simulink model "visual_servoing"  (R2023a)
settings: Solver=ode2  StartTime=0.0  StopTime=inf  FixedStep=1/30  RelTol=1e-3  EnableMultiTasking=on
undefined symbols (not defined in the file): gcbh, height, HIL, JPEG, left, qc_get_step_size, top, video_display_show, width
libraries: quarc_library x21, simulink x4
settings Model: ExtModeTrigDuration=10000  Creator=msaravanan  LastModifiedBy=msaravanan
settings SolverCC: AlgebraicLoopSolver=TrustRegion  PositivePriorityOrder=on
settings DataIOCC: ReturnWorkspaceOutputs=off
settings DebuggingCC: UnconnectedInputMsg=warning  UnconnectedOutputMsg=warning  UnconnectedLineMsg=warning  ArithmeticOperatorsInVariantConditions=warning
settings ModelReferenceCC: EnableRefExpFcnMdlSchedulingChecks=on
settings SFSimCC: SimUseLocalCustomCode=off  CustomCodeUndefinedFunction=UseInterfaceOnly
settings RTWCC: Description=QUARC Win64 Target Using Toolchain  SystemTargetFile=quarc_win64.tlc  TemplateMakefile=quarc_default_tmf  RTWUseLocalCustomCode=off  Toolchain=QUARC win64 | nmake (64-bit Windows)  BuildConfiguration=Faster Runs
settings CodeAppCC: StateflowObjectComments=on
settings STFCustomTargetCC: SystemTargetFile=quarc_win64.tlc
settings GRTTargetCC: ParMdlRefBuildCompliant=off  CompOptLevelCompliant=off  CombineOutputUpdateFcns=off  MatFileLogging=off  CPPClassGenCompliant=off  GRTInterface=on  ExtMode=on  ExtModeMexFile=quarc_comm
settings ConfigComp: CovMetricSettings=dswe

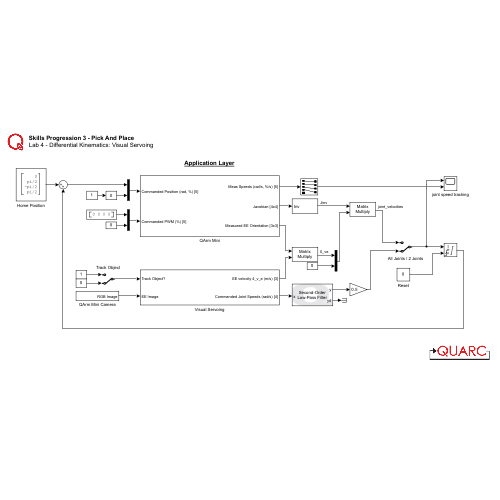
[thumbnail: Simulink's stored preview of the top-level diagram]
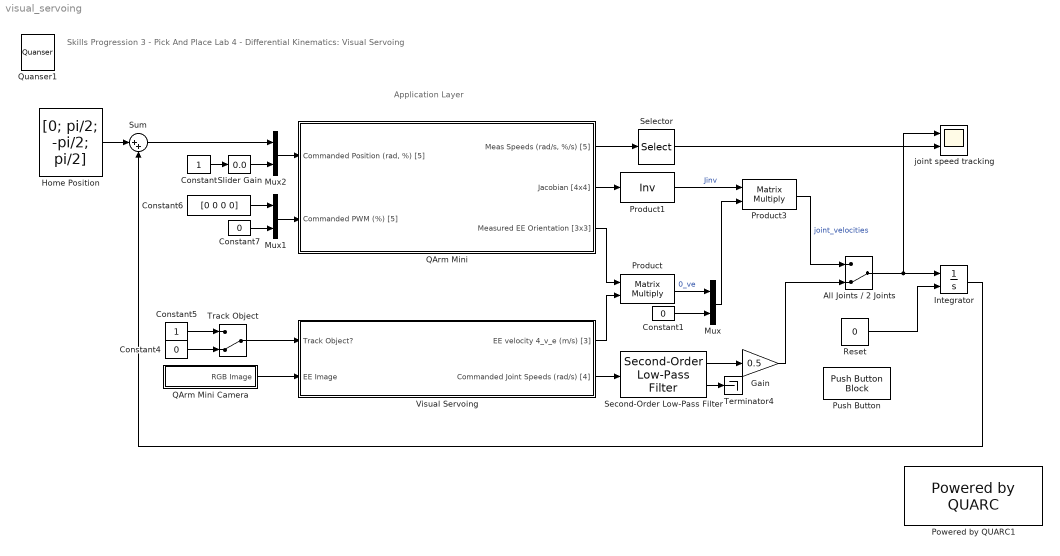
== system visual_servoing ==
  note: Skills Progression 3 - Pick And Place
      | Lab 4 - Differential Kinematics: Visual Servoing
  note: Application Layer
  All Joints / 2 Joints : ManualSwitch  CurrentSetting=0
  Constant : Constant
  Constant1 : Constant  Value=0
  Constant4 : Constant  Value=0
  Constant5 : Constant
  Constant6 : Constant  Value=[0 0 0 0]
  Constant7 : Constant  Value=0
  Gain : Gain  Gain=0.5
  Home Position : Constant  Value=[0; pi/2; -pi/2; pi/2]  VectorParams1D=off
  Integrator : Integrator  ExternalReset=rising  InitialCondition=[0; 0; 0; 0]  LimitOutput=on  UpperSaturationLimit=2*[pi/6; pi/6; pi/6; pi/6]  LowerSaturationLimit=-2*[pi/6; pi/6; pi/6; pi/6]
  Mux : Mux  Inputs=2
  Mux1 : Mux  Inputs=2
  Mux2 : Mux  Inputs=2
  Powered by QUARC1 : quarc_library/Logos/Powered by QUARC
  Product : Product  Multiplication=Matrix(*)
  Product1 : Product  Inputs=/  Multiplication=Matrix(*)
  Product3 : Product  Multiplication=Matrix(*)
  Push Button : PushButtonBlock  ButtonText=Reset  OffValue=0.000000
  QArm Mini : Subsystem
  QArm Mini Camera : Subsystem
  Quanser1 : quarc_library/Logos/Quanser
  Reset : Constant  Value=0
  Second-Order Low-Pass Filter : quarc_library/Continuous/Second-Order Low-Pass Filter  params_source=Internal (dialog parameters)  input_width=5  input_zeta=1  input_init=0
  Selector : Selector  InputPortWidth=5  IndexOptions=Index vector (dialog)  Indices=[1:4]  OutputSizes=1
  Slider Gain : simulink/Math Operations/Slider Gain  gain=0.0  low=0  high=1
  Sum : Sum  Inputs=|++
  Terminator4 : Terminator
  Track Object : ManualSwitch  CurrentSetting=0
  Visual Servoing : Subsystem
  joint speed tracking : Scope  NumInputPorts=2
  wires:
  Visual Servoing/1(EE velocity 4_v_e (m/s) [3]) -> Product/2
  Product/1 -> Mux/1  "0_ve"
  Constant1/1 -> Mux/2
  Mux/1 -> Product3/2
  Product3/1 -> All Joints / 2 Joints/1  "joint_velocities"
  Track Object/1 -> Visual Servoing/1(Track Object?)
  All Joints / 2 Joints/1 -> joint speed tracking/1, Integrator/1
  Reset/1 -> Integrator/2
  Visual Servoing/2(Commanded Joint Speeds (rad/s) [4]) -> Second-Order Low-Pass Filter/1
  Second-Order Low-Pass Filter/1 -> Gain/1
  Second-Order Low-Pass Filter/2 -> Terminator4/1
  Home Position/1 -> Sum/1
  Mux2/1 -> QArm Mini/1("Commanded Position (rad, %) [5]")
  Mux1/1 -> QArm Mini/2(Commanded PWM (%) [5])
  Constant7/1 -> Mux1/2
  Slider Gain/1 -> Mux2/2
  Sum/1 -> Mux2/1
  Constant/1 -> Slider Gain/1
  Constant6/1 -> Mux1/1
  Integrator/1 -> Sum/2
  Constant4/1 -> Track Object/2
  Constant5/1 -> Track Object/1
  QArm Mini/3(Measured EE Orientation [3x3]) -> Product/1
  QArm Mini/2(Jacobian [4x4]) -> Product1/1
  Gain/1 -> All Joints / 2 Joints/2
  Product1/1 -> Product3/1  "Jinv"
  QArm Mini/1("Meas Speeds (rad/s, %/s) [5]") -> Selector/1
  Selector/1 -> joint speed tracking/2
  QArm Mini Camera/1(RGB Image) -> Visual Servoing/2(EE Image)

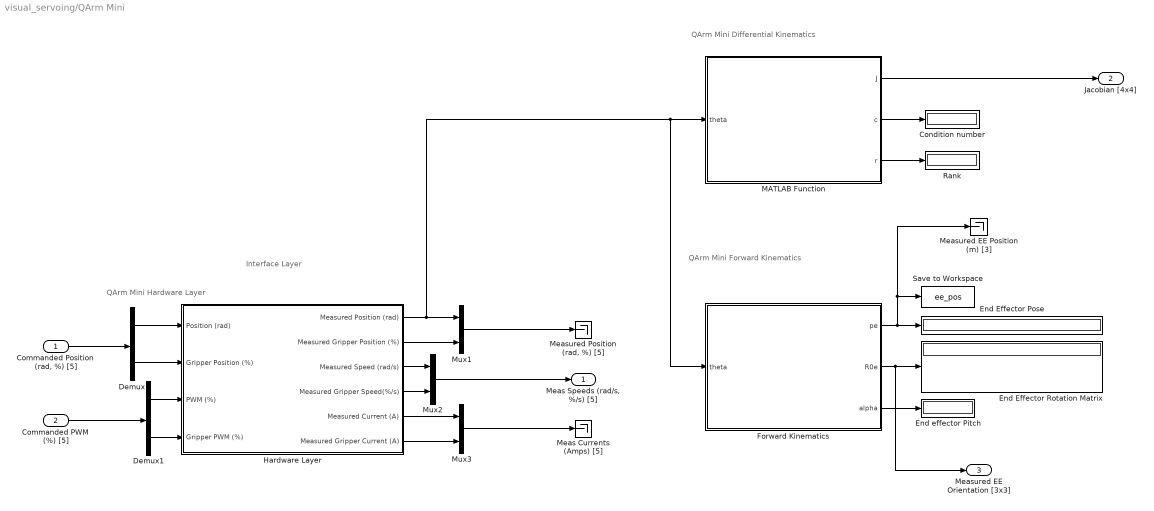
== system visual_servoing/QArm Mini ==
  note: QArm Mini Forward Kinematics
  note: Interface Layer
  note: QArm Mini Hardware Layer
  note: QArm Mini Differential Kinematics
  "Commanded Position (rad, %) [5]" : Inport
  Commanded PWM (%) [5] : Inport  Port=2
  Condition number : Display
  Demux : Demux  Outputs=[4 1]
  Demux1 : Demux  Outputs=[4 1]
  End Effector Pose : Display
  End Effector Rotation Matrix : Display
  End effector Pitch : Display
  Forward Kinematics : MATLAB Function  TreatAsAtomicUnit=on
  Hardware Layer : Subsystem
  MATLAB Function : MATLAB Function  TreatAsAtomicUnit=on
  Meas Currents (Amps) [5] : Terminator
  Measured EE Position (m) [3] : Terminator
  "Measured Position (rad, %) [5]" : Terminator
  Mux1 : Mux  Inputs=2
  Mux2 : Mux  Inputs=2
  Mux3 : Mux  Inputs=2
  Rank : Display
  Save to Workspace : ToWorkspace  VariableName=ee_pos  SaveFormat=Structure With Time  SampleTime=-1
  "Meas Speeds (rad/s, %/s) [5]" : Outport
  Jacobian [4x4] : Outport  Port=2
  Measured EE Orientation [3x3] : Outport  Port=3
  wires:
  Demux/2 -> Hardware Layer/2(Gripper Position (%))
  Hardware Layer/1(Measured Position (rad)) -> Mux1/1, Forward Kinematics/1(theta), MATLAB Function/1(theta)
  Forward Kinematics/2(R0e) -> Measured EE Orientation [3x3]/1, End Effector Rotation Matrix/1
  Forward Kinematics/3(alpha) -> End effector Pitch/1
  Demux1/2 -> Hardware Layer/4(Gripper PWM (%))
  Hardware Layer/2(Measured Gripper Position (%)) -> Mux1/2
  Hardware Layer/3(Measured Speed (rad/s)) -> Mux2/1
  Hardware Layer/4(Measured Gripper Speed(%/s)) -> Mux2/2
  Hardware Layer/5(Measured Current (A)) -> Mux3/1
  Hardware Layer/6(Measured Gripper Current (A)) -> Mux3/2
  Mux3/1 -> Meas Currents (Amps) [5]/1
  Mux2/1 -> "Meas Speeds (rad/s, %/s) [5]"/1
  Mux1/1 -> "Measured Position (rad, %) [5]"/1
  "Commanded Position (rad, %) [5]"/1 -> Demux/1
  Demux/1 -> Hardware Layer/1(Position (rad))
  Demux1/1 -> Hardware Layer/3(PWM (%))
  Commanded PWM (%) [5]/1 -> Demux1/1
  Forward Kinematics/1(pe) -> Measured EE Position (m) [3]/1, Save to Workspace/1, End Effector Pose/1
  MATLAB Function/3(r) -> Rank/1
  MATLAB Function/2(c) -> Condition number/1
  MATLAB Function/1(J) -> Jacobian [4x4]/1

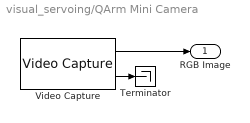
== system visual_servoing/QArm Mini Camera ==
  Terminator : Terminator
  Video Capture : quarc_library/Multimedia/Video Capture  source=device  device=0  filename=sample_movie.mov  value=[0 0; 0 0]  resolution=1280 x 720  width=1280  height=720  output_format=MATLAB RGB (HxWx3)  data_type=uint8  sample_time=qc_get_step_size * ceil(0.033 / qc_get_step_size)  brightness_override=Do not override  brightness=50.0  contrast_override=Do not override  contrast=50.0  hue_override=Do not override  hue=50.0  saturation_override=Do not override  saturation=50.0  sharpness_override=Do not override  sharpness=50.0  gamma_override=Do not override  gamma=50.0  coloreffect_override=Do not override  coloreffect=None  whitebalance_override=Do not override  whitebalance=50.0  backlightcompensation_override=Do not override  backlightcompensation=0.0  gain_override=Do not override  gain=50.0  pan_override=Do not override  pan=50.0  tilt_override=Do not override  tilt=50.0  roll_override=Do not override  roll=50.0  zoom_override=Do not override  zoom=0.0  exposure_override=Do not override  exposure=50.0  iris_override=Do not override  iris=50.0  mirror_override=Do not override  mirror=None  focus_override=Do not override  focus=0.0
      settings: SourceProductName=QUARC Targets
  RGB Image : Outport
  wires:
  Video Capture/2 -> Terminator/1
  Video Capture/1 -> RGB Image/1

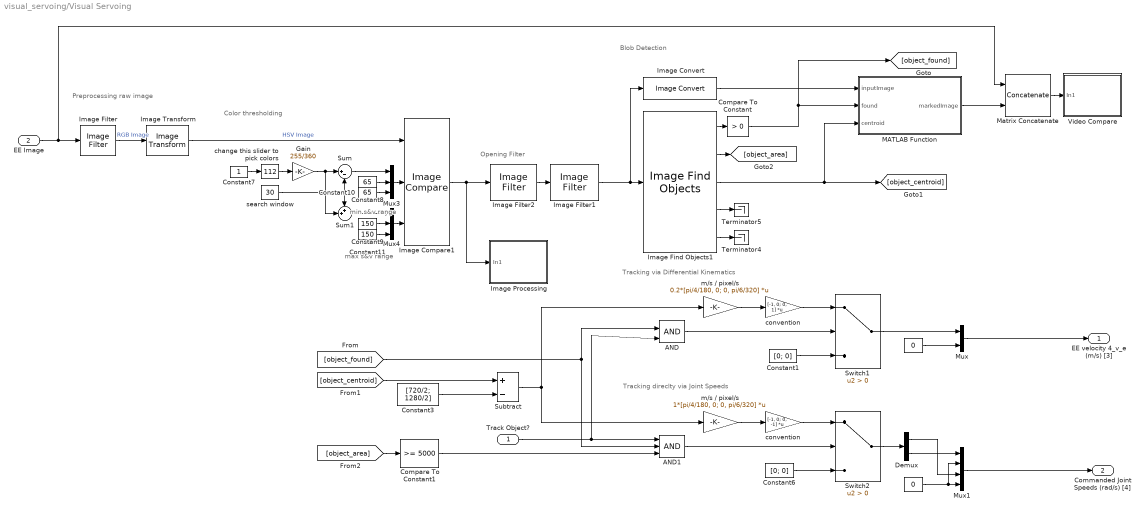
== system visual_servoing/Visual Servoing ==
  note: max s&v range
  note: min s&v range
  note: Tracking via Differential Kinematics
  note: Color thresholding
  note: Opening Filter
  note: Preprocessing raw image
  note: Blob Detection
  note: Tracking direclty via Joint Speeds
  Track Object? : Inport
  EE Image : Inport  Port=2
  " " : Constant  Value=0
  "    " : Constant  Value=0
  " convention " : Gain  Gain=[-1, 0; 0, -1]  Multiplication=Matrix(K*u)
  " m/s / pixel/s " : Gain  Gain=1*[pi/4/180, 0; 0, pi/6/320]  Multiplication=Matrix(K*u)
  AND : Logic  IconShape=distinctive  AllPortsSameDT=off  OutDataTypeStr=boolean
  AND1 : Logic  Inputs=3  IconShape=distinctive  AllPortsSameDT=off  OutDataTypeStr=boolean
  Compare To Constant : simulink/Logic and Bit Operations/Compare To Constant  relop=>  const=0  OutDataTypeStr=boolean
  Compare To Constant1 : simulink/Logic and Bit Operations/Compare To Constant  relop=>=  const=5000  OutDataTypeStr=boolean
  Constant1 : Constant  Value=[0; 0]
  Constant10 : Constant  Value=65
  Constant11 : Constant  Value=150
  Constant3 : Constant  Value=[720/2; 1280/2]  VectorParams1D=off
  Constant6 : Constant  Value=[0; 0]
  Constant7 : Constant
  Constant8 : Constant  Value=65
  Constant9 : Constant  Value=150
  Demux : Demux  Outputs=2
  Gain : Gain  Gain=255/360
  Image Compare1 : quarc_library/Image Processing/Generic/Image Compare  output_type=Combined (one HxW output)  source=External input ports  r_comparison=min <= pixel and pixel <= max with wrapping  r_minimum=0  r_maximum=10  g_comparison=min <= pixel and pixel <= max with wrapping  g_minimum=0  g_maximum=64  b_comparison=min <= pixel and pixel <= max with wrapping  b_minimum=0  b_maximum=200
      settings: SourceProductName=QUARC Targets
  Image Convert : quarc_library/Image Processing/Generic/Image Convert  input_format=MATLAB greyscale (HxW)  padding=0  output_format=MATLAB RGB (HxWx3)  data_type=uint8
      settings: AttributesFormatString=(%<input_format>)  SourceProductName=QUARC Targets
  Image Filter : quarc_library/Image Processing/Generic/Image Filter  filter_type=Gaussian  source_of_roi=Internal dialog parameter  roi_style=[top, left, height, width]  roi=[]  maximum_roi=[]  roi_zone=Operate inside region of interest  border_type=Replicate  border_value=[0 0 0]  kernel_size=5  sigma=1  mask_size=[3 3]  kernel=int16([-2 -1 0; -1 1 1; 0 1 2])  divisor=1  offset=0  rounding=Nearest  algorithm_hint=None  threshold=100  alpha=0.9  num_frames=8  num_valid=1  gap_threshold=10  depth_threshold=255  iterations=2  norm_type=L1
      settings: AttributesFormatString=(%<filter_type>)  SourceProductName=QUARC Targets
  Image Filter1 : quarc_library/Image Processing/Generic/Image Filter  filter_type=Maximum  source_of_roi=Internal dialog parameter  roi_style=[top, left, height, width]  roi=[]  maximum_roi=[]  roi_zone=Operate inside region of interest  border_type=Replicate  border_value=[0 0 0]  kernel_size=15  sigma=.2  mask_size=[5 5]  kernel=int16([-2 -1 0; -1 1 1; 0 1 2])  divisor=1  offset=0  rounding=Nearest  algorithm_hint=None  threshold=100  alpha=0.9  num_frames=8  num_valid=1  gap_threshold=10  depth_threshold=255  iterations=2  norm_type=L1
      settings: AttributesFormatString=(%<filter_type>)  SourceProductName=QUARC Targets
  Image Filter2 : quarc_library/Image Processing/Generic/Image Filter  filter_type=Minimum  source_of_roi=Internal dialog parameter  roi_style=[top, left, height, width]  roi=[]  maximum_roi=[]  roi_zone=Operate inside region of interest  border_type=Replicate  border_value=[0 0 0]  kernel_size=15  sigma=.2  mask_size=[5 5]  kernel=int16([-2 -1 0; -1 1 1; 0 1 2])  divisor=1  offset=0  rounding=Nearest  algorithm_hint=None  threshold=100  alpha=0.9  num_frames=8  num_valid=1  gap_threshold=10  depth_threshold=255  iterations=2  norm_type=L1
      settings: AttributesFormatString=(%<filter_type>)  SourceProductName=QUARC Targets
  Image Find Objects1 : quarc_library/Image Processing/Generic/Image Find Objects  num_objects=1  connectivity=8 directions (N, NE, E, SE, S, SW, W, NW)  sort_order=Sort by number of pixels  min_pixels=500  max_pixels=intmax('uint32')  largest=on  exclude_at_edges=off  variable_size=off  use_complex=off
      settings: SourceProductName=QUARC Targets
  Image Processing : Subsystem  LoadFcn=set_param(gcbh, 'UserData', gcb);  StartFcn=video_display_show([gcb, '/Video Display'], 'add', gcb);  mask(Video Compressed Display){algorithm=JPEG, quality=50, sample_time=-1, use_hardware=on}
      mask prompts: algorithm "Compression algorithm:"; quality "Compression quality (0-100):"; sample_time "Sample time (seconds):"; use_hardware "Use hardware acceleration for video display"
      mask help: Displays a video stream on the host, using compression to minimize bandwidth.
      mask init:
      | qc_set_display('Video\nCompressed\nDisplay');
      settings: UndoDeleteFcn=set_param(gcbh, 'UserData', gcb);  OpenFcn=video_display_show([gcb, '/Video Display'], 'show', gcb);  PreDeleteFcn=video_display_show([gcb, '/Video Display'], 'delete');
      settings: CopyFcn=|
      | set_param(gcbh, 'UserData', gcb);
      | set_param(gcbh, 'LinkStatus', 'none');
      settings: NameChangeFcn=|
      | video_display_show([get_param(gcbh, 'UserData'), '/Video Display'], 'rename', [gcb, '/Video Display']);
      | video_display_show([gcb, '/Video Display'], 'add', gcb);
      | set_param(gcbh, 'UserData', gcb);
      mask Help: web(qc_get_block_help_path(gcb));
      mask TypeOptions algorithm: Image Compress/algorithm
      mask TypeOptions quality: Image Compress/quality
      mask TypeOptions sample_time: Video Display/sample_time
      mask TypeOptions use_hardware: Video Display/use_hardware
      mask Display:
      | patch([0.98591 0.98591 0.62618 0.59072 0.56147   0.536   0.536  0.5441 0.56912 0.59207 0.60881 0.62276 0.63527 0.64364  0.6485  0.6485 0.64706 0.64499 0.63662 0.62411 0.61232 0.59837 0.58307 0.56147   0.536   0.536  0.5441  0.5747 0.60953 0.63662 0.67001  0.7034 0.72851 0.75425 0.77927 0.80294 0.82454 0.84119 0.85865 0.87395 0.88574 0.89339  0.8969 0.89969 0.89969 0.89267  0.8816 0.87044 0.85649  0.8384 0.81824 0.80294 0.78764 0.77513 0.76676 0.75776 0.76397 0.77513 0.79178 0.80987 0.82796 0.84326 0.86207 0.98528],[0.18689 0.05522 0.05522 0.05171 0.05171    0.05 0.18338 0.18338 0.19148 0.20435 0.22298 0.24863 0.28589 0.33125 0.38138 0.55139 0.59801 0.63761 0.68189 0.72149 0.74939 0.76694 0.77855 0.79367 0.79952 0.92768 0.92768 0.92768 0.92417 0.92066 0.91364  0.9032 0.89384 0.88106 0.86594 0.85073 0.82634 0.80537 0.77855 0.74363 0.70403 0.65858 0.61079 0.59099 0.41513 0.37202 0.31847 0.29048 0.25556 0.23342  0.2102 0.19382 0.18221 0.17285 0.16943 0.16124  0.1589 0.16241 0.16709 0.17168  0.1787 0.18221 0.18689 0.18689],[0.9,0.90,0.91])
      | patch([0.536 0.52601 0.46823 0.44528 0.41603 0.39101 0.35555 0.33116 0.31451 0.29291  0.2804 0.26717 0.25322 0.23999 0.22406 0.20732 0.19337 0.17528 0.15935 0.14396 0.13217 0.11759 0.10922 0.10085 0.09671 0.09392 0.09041 0.08906 0.08906 0.09464  0.0995 0.10778 0.11894 0.13145 0.14675 0.16349 0.17672 0.19409 0.20732 0.22406 0.23999 0.26159 0.27833 0.29849 0.31793 0.33602 0.35411 0.37085 0.39245 0.41603   0.536   0.536 0.53159 0.46409   0.446 0.42026 0.39587 0.37571 0.36113 0.34925 0.34088 0.33809 0.33809 0.34088 0.34583 0.35627 0.36392 0.38129 0.39587 0.41117 0.42719 0.44672  0.4676 0.48353 0.48353 0.52394   0.536],[0.05 0.04829 0.04712 0.04712 0.04829 0.05063 0.05405 0.05873 0.06107 0.06692 0.07043 0.07619 0.08087 0.08672 0.09482 0.10652 0.11696 0.13325  0.1508 0.17168 0.19499 0.22415 0.25439 0.28472 0.31379 0.35456 0.38489 0.41513 0.58055 0.63878 0.68774 0.72149 0.75641 0.78089 0.80537 0.82859 0.84029 0.85658 0.86594 0.87404  0.8834 0.89267 0.90086 0.90788 0.91247 0.91832 0.92066   0.923 0.92651 0.92768 0.92768 0.79952 0.79952 0.79952 0.79718 0.78899 0.77153 0.75056 0.72149 0.68072 0.62249  0.5549 0.41396 0.37085 0.33242 0.28121 0.25205 0.22181 0.20552 0.19499 0.18572 0.18221 0.17753 0.17636 0.17753  0.1787  0.1787],[0.9,0.90,0.91])
      | disp('Video\nCompressed\nDisplay');
  Image Transform : quarc_library/Image Processing/Generic/Image Transform  algorithm=RGB to HSV  color_theme=KRYGCBMW  min_pixel=0  max_pixel=4000  contour_depth=1  focal_length=308  principal_point=[262 334]  radial_coeffs=[-0.3129 0.0907]  tangential_coeffs=[]  extrapolated_pixel=0  interpolation=nearest  row_coords=0  column_coords=0  output_height=480  output_width=640  angle=0  origin=[240 320]  output_origin=[240 320]  output_data_type=uint8
      settings: AttributesFormatString=(%<algorithm>)  SourceProductName=QUARC Targets
  MATLAB Function : MATLAB Function  TreatAsAtomicUnit=on
  Matrix Concatenate : Concatenate  Mode=Multidimensional array  ConcatenateDimension=2
  Mux : Mux  Inputs=2
  Mux1 : Mux
  Mux3 : Mux  Inputs=3
  Mux4 : Mux  Inputs=3
  Subtract : Sum  Inputs=+-
  Sum : Sum  Inputs=|+-
  Sum1 : Sum  Inputs=++|
  Switch1 : Switch  Criteria=u2 > Threshold  SaturateOnIntegerOverflow=off  InputSameDT=off
  Switch2 : Switch  Criteria=u2 > Threshold  SaturateOnIntegerOverflow=off  InputSameDT=off
  Terminator4 : Terminator
  Terminator5 : Terminator
  Video Compare : Subsystem  LoadFcn=set_param(gcbh, 'UserData', gcb);  StartFcn=video_display_show([gcb, '/Video Display'], 'add', gcb);  mask(Video Compressed Display){algorithm=JPEG, quality=50, sample_time=-1, use_hardware=on}
      mask prompts: algorithm "Compression algorithm:"; quality "Compression quality (0-100):"; sample_time "Sample time (seconds):"; use_hardware "Use hardware acceleration for video display"
      mask help: Displays a video stream on the host, using compression to minimize bandwidth.
      mask init:
      | qc_set_display('Video\nCompressed\nDisplay');
      settings: UndoDeleteFcn=set_param(gcbh, 'UserData', gcb);  OpenFcn=video_display_show([gcb, '/Video Display'], 'show', gcb);  PreDeleteFcn=video_display_show([gcb, '/Video Display'], 'delete');
      settings: CopyFcn=|
      | set_param(gcbh, 'UserData', gcb);
      | set_param(gcbh, 'LinkStatus', 'none');
      settings: NameChangeFcn=|
      | video_display_show([get_param(gcbh, 'UserData'), '/Video Display'], 'rename', [gcb, '/Video Display']);
      | video_display_show([gcb, '/Video Display'], 'add', gcb);
      | set_param(gcbh, 'UserData', gcb);
      mask Help: web(qc_get_block_help_path(gcb));
      mask TypeOptions algorithm: Image Compress/algorithm
      mask TypeOptions quality: Image Compress/quality
      mask TypeOptions sample_time: Video Display/sample_time
      mask TypeOptions use_hardware: Video Display/use_hardware
      mask Display:
      | patch([0.98591 0.98591 0.62618 0.59072 0.56147   0.536   0.536  0.5441 0.56912 0.59207 0.60881 0.62276 0.63527 0.64364  0.6485  0.6485 0.64706 0.64499 0.63662 0.62411 0.61232 0.59837 0.58307 0.56147   0.536   0.536  0.5441  0.5747 0.60953 0.63662 0.67001  0.7034 0.72851 0.75425 0.77927 0.80294 0.82454 0.84119 0.85865 0.87395 0.88574 0.89339  0.8969 0.89969 0.89969 0.89267  0.8816 0.87044 0.85649  0.8384 0.81824 0.80294 0.78764 0.77513 0.76676 0.75776 0.76397 0.77513 0.79178 0.80987 0.82796 0.84326 0.86207 0.98528],[0.18689 0.05522 0.05522 0.05171 0.05171    0.05 0.18338 0.18338 0.19148 0.20435 0.22298 0.24863 0.28589 0.33125 0.38138 0.55139 0.59801 0.63761 0.68189 0.72149 0.74939 0.76694 0.77855 0.79367 0.79952 0.92768 0.92768 0.92768 0.92417 0.92066 0.91364  0.9032 0.89384 0.88106 0.86594 0.85073 0.82634 0.80537 0.77855 0.74363 0.70403 0.65858 0.61079 0.59099 0.41513 0.37202 0.31847 0.29048 0.25556 0.23342  0.2102 0.19382 0.18221 0.17285 0.16943 0.16124  0.1589 0.16241 0.16709 0.17168  0.1787 0.18221 0.18689 0.18689],[0.9,0.90,0.91])
      | patch([0.536 0.52601 0.46823 0.44528 0.41603 0.39101 0.35555 0.33116 0.31451 0.29291  0.2804 0.26717 0.25322 0.23999 0.22406 0.20732 0.19337 0.17528 0.15935 0.14396 0.13217 0.11759 0.10922 0.10085 0.09671 0.09392 0.09041 0.08906 0.08906 0.09464  0.0995 0.10778 0.11894 0.13145 0.14675 0.16349 0.17672 0.19409 0.20732 0.22406 0.23999 0.26159 0.27833 0.29849 0.31793 0.33602 0.35411 0.37085 0.39245 0.41603   0.536   0.536 0.53159 0.46409   0.446 0.42026 0.39587 0.37571 0.36113 0.34925 0.34088 0.33809 0.33809 0.34088 0.34583 0.35627 0.36392 0.38129 0.39587 0.41117 0.42719 0.44672  0.4676 0.48353 0.48353 0.52394   0.536],[0.05 0.04829 0.04712 0.04712 0.04829 0.05063 0.05405 0.05873 0.06107 0.06692 0.07043 0.07619 0.08087 0.08672 0.09482 0.10652 0.11696 0.13325  0.1508 0.17168 0.19499 0.22415 0.25439 0.28472 0.31379 0.35456 0.38489 0.41513 0.58055 0.63878 0.68774 0.72149 0.75641 0.78089 0.80537 0.82859 0.84029 0.85658 0.86594 0.87404  0.8834 0.89267 0.90086 0.90788 0.91247 0.91832 0.92066   0.923 0.92651 0.92768 0.92768 0.79952 0.79952 0.79952 0.79718 0.78899 0.77153 0.75056 0.72149 0.68072 0.62249  0.5549 0.41396 0.37085 0.33242 0.28121 0.25205 0.22181 0.20552 0.19499 0.18572 0.18221 0.17753 0.17636 0.17753  0.1787  0.1787],[0.9,0.90,0.91])
      | disp('Video\nCompressed\nDisplay');
  change this slider to pick colors : simulink/Math Operations/Slider Gain  gain=112  low=0  high=360
  convention : Gain  Gain=[-1, 0; 0, 1]  Multiplication=Matrix(K*u)
  m/s / pixel/s : Gain  Gain=0.2*[pi/4/180, 0; 0, pi/6/320]  Multiplication=Matrix(K*u)
  search window : Constant  Value=30
  EE velocity 4_v_e (m/s) [3] : Outport
  Commanded Joint Speeds (rad/s) [4] : Outport  Port=2
  wires:
  Subtract/1 -> " m/s / pixel/s "/1, m/s / pixel/s/1
  EE Image/1 -> Matrix Concatenate/1, Image Filter/1
  MATLAB Function/1(markedImage) -> Matrix Concatenate/2
  Image Convert/1 -> MATLAB Function/1(inputImage)
  m/s / pixel/s/1 -> convention/1
  Image Filter2/1 -> Image Filter1/1
  [object_centroid] -> Subtract/1
  Image Filter1/1 -> Image Convert/1, Image Find Objects1/1
  Image Find Objects1/1 -> Compare To Constant/1
  Sum/1 -> Mux3/1
  Constant10/1 -> Mux3/3
  Matrix Concatenate/1 -> Video Compare/1(In1)
  search window/1 -> Sum1/1, Sum/2
  Gain/1 -> Sum1/2, Sum/1
  Constant7/1 -> change this slider to pick colors/1
  Switch1/1 -> Mux/1
  Constant11/1 -> Mux4/3
  Mux/1 -> EE velocity 4_v_e (m/s) [3]/1
  Image Find Objects1/5 -> Terminator4/1
  Sum1/1 -> Mux4/1
  Image Find Objects1/4 -> Terminator5/1
  Image Filter/1 -> Image Transform/1  "RGB Image"
  "    "/1 -> Mux/2
  Mux4/1 -> Image Compare1/3
  Image Transform/1 -> Image Compare1/1  "HSV Image"
  Mux3/1 -> Image Compare1/2
  change this slider to pick colors/1 -> Gain/1
  Image Compare1/1 -> Image Filter2/1, Image Processing/1(In1)
  Constant8/1 -> Mux3/2
  Constant9/1 -> Mux4/2
  Constant3/1 -> Subtract/2
  convention/1 -> Switch1/1
  Constant1/1 -> Switch1/3
  AND/1 -> Switch1/2
  AND1/1 -> Switch2/2
  Track Object?/1 -> AND/2, AND1/1
  Constant6/1 -> Switch2/3
  " m/s / pixel/s "/1 -> " convention "/1
  Mux1/1 -> Commanded Joint Speeds (rad/s) [4]/1
  " convention "/1 -> Switch2/1
  Demux/2 -> Mux1/1
  Demux/1 -> Mux1/3
  " "/1 -> Mux1/4, Mux1/2
  Compare To Constant1/1 -> AND1/3
  Switch2/1 -> Demux/1
  Compare To Constant/1 -> [object_found], MATLAB Function/2(found)
  [object_found] -> AND1/2, AND/1
  Image Find Objects1/3 -> MATLAB Function/3(centroid), [object_centroid]
  Image Find Objects1/2 -> [object_area]
  [object_area] -> Compare To Constant1/1

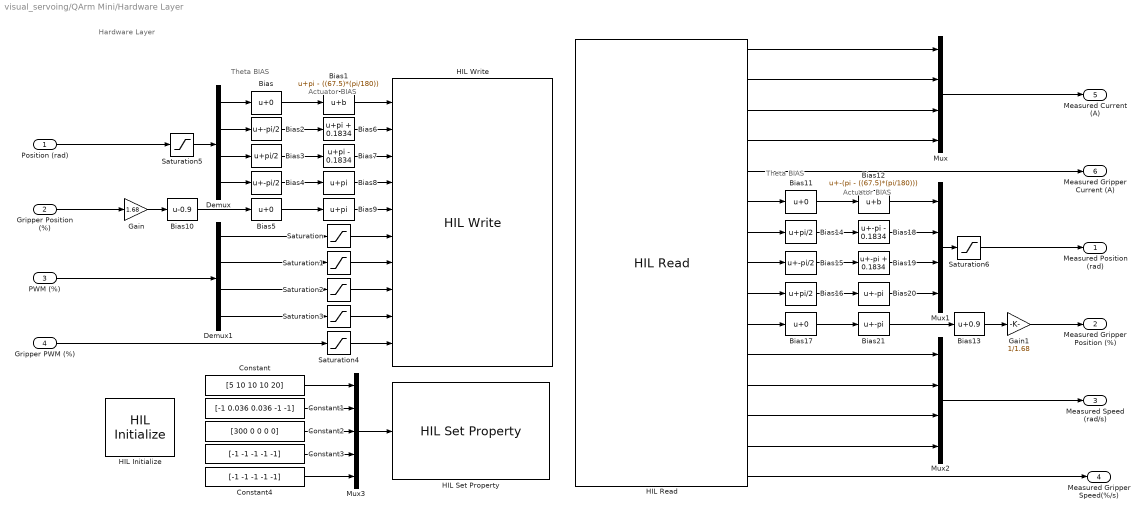
== system visual_servoing/QArm Mini/Hardware Layer ==
  note: Hardware Layer
  note: Actuator BIAS
  note: Theta BIAS
  note: Actuator BIAS
  note: Theta BIAS
  Position (rad) : Inport
  Gripper Position (%) : Inport  Port=2
  PWM (%) : Inport  Port=3
  Gripper PWM (%) : Inport  Port=4
  Bias{,5,11,17} (4 alike) : Bias  SaturateOnIntegerOverflow=off
  Bias1 : Bias  Bias=pi - ((67.5)*(pi/180))  SaturateOnIntegerOverflow=off
  Bias10 : Bias  Bias=-0.9  SaturateOnIntegerOverflow=off
  Bias12 : Bias  Bias=-(pi - ((67.5)*(pi/180)))  SaturateOnIntegerOverflow=off
  Bias13 : Bias  Bias=0.9  SaturateOnIntegerOverflow=off
  Bias14 : Bias  Bias=pi/2  SaturateOnIntegerOverflow=off
  Bias15 : Bias  Bias=-pi/2  SaturateOnIntegerOverflow=off
  Bias16 : Bias  Bias=pi/2  SaturateOnIntegerOverflow=off
  Bias18 : Bias  Bias="-pi -  0.1834"  SaturateOnIntegerOverflow=off
  Bias19 : Bias  Bias="-pi +  0.1834"  SaturateOnIntegerOverflow=off
  Bias2 : Bias  Bias=-pi/2  SaturateOnIntegerOverflow=off
  Bias20 : Bias  Bias=-pi  SaturateOnIntegerOverflow=off
  Bias21 : Bias  Bias=-pi  SaturateOnIntegerOverflow=off
  Bias3 : Bias  Bias=pi/2  SaturateOnIntegerOverflow=off
  Bias4 : Bias  Bias=-pi/2  SaturateOnIntegerOverflow=off
  Bias6 : Bias  Bias=pi + 0.1834  SaturateOnIntegerOverflow=off
  Bias7 : Bias  Bias="pi -  0.1834"  SaturateOnIntegerOverflow=off
  Bias8 : Bias  Bias=pi  SaturateOnIntegerOverflow=off
  Bias9 : Bias  Bias=pi  SaturateOnIntegerOverflow=off
  Constant : Constant  Value=[5 10 10 10 20]
  Constant1 : Constant  Value=[-1 0.036 0.036 -1 -1]
  Constant2 : Constant  Value=[300 0 0 0 0]
  Constant3 : Constant  Value=[-1 -1 -1 -1 -1]
  Constant4 : Constant  Value=[-1 -1 -1 -1 -1]
  Demux : Demux
  Demux1 : Demux
  Gain : Gain  Gain=1.68
  Gain1 : Gain  Gain=1/1.68
  "HIL Initialize " : quarc_library/Data Acquisition/Generic/Configuration/HIL Initialize  object_name=HIL-1  board_type=qarm_mini  board_number=7  board_options=j0_mode=0;j1_mode=0;j2_mode=0;j3_mode=0;gripper_mode=0;j0_profile_velocity=6.2832;j0_profile_acceleration=6.2832;j1_profile_velocity=6.2832;j1_profile_acceleration=6.2832;j2_profile_velocity=6.2832;j2_profile_acceleration=6.2832;j3_profile_velocity=6.2832;j3_profile_acceleration=6.2832;gripper_profile_velocity=6.2832;gripper_profile_acceleration=6.2832;  exclusive=off  active=on  hardware_clocks=[]  clock_modes=[]  initial_clock_frequencies=[]  set_clock_params_at_start=off  set_clock_params_at_switch_in=off  set_clock_frequencies_at_start=off  set_clock_frequencies_at_switch_in=off  analog_input_channels=[0:4]  analog_input_configurations=[]  analog_input_maximums=[100 3.21 3.21 3.21 100]  analog_input_minimums=[-100 -3.21 -3.21 -3.21 -100]  set_analog_input_params_at_start=off  set_analog_input_params_at_switch_in=off  analog_output_channels=[]  analog_output_maximums=[]  analog_output_minimums=[]  initial_analog_outputs=[]  final_analog_outputs=[]  watchdog_analog_outputs=[]  set_analog_output_params_at_start=off  set_analog_output_params_at_switch_in=off  set_analog_outputs_at_start=off  set_analog_outputs_at_switch_in=off  set_analog_outputs_at_terminate=off  set_analog_outputs_at_switch_out=off  set_analog_outputs_on_watchdog=off  digital_input_channels=[]  digital_output_channels=[]  digital_output_configuration=[]  initial_digital_outputs=[]  final_digital_outputs=[]  watchdog_digital_outputs=[]  set_digital_output_params_at_start=off  set_digital_output_params_at_switch_in=off  set_digital_outputs_at_start=off  set_digital_outputs_at_switch_in=off  set_digital_outputs_at_terminate=off  set_digital_outputs_at_switch_out=off  set_digital_outputs_on_watchdog=off  encoder_channels=[]  quadrature=[]  encoder_filter_frequency=[]  initial_encoder_counts=[]  set_encoder_params_at_start=off  set_encoder_params_at_switch_in=off  set_encoder_counts_at_start=off  set_encoder_counts_at_switch_in=off  pwm_channels=[]  pwm_modes=[]  pwm_frequency=[]  pwm_configuration=[]  pwm_alignment=[]  pwm_polarity=[]  pwm_leading_deadband=[]  pwm_trailing_deadband=[]  initial_pwm_outputs=[]  final_pwm_outputs=[]  watchdog_pwm_outputs=[]  set_pwm_params_at_start=off  set_pwm_params_at_switch_in=off  set_pwm_outputs_at_start=off  set_pwm_outputs_at_switch_in=off  set_pwm_outputs_at_terminate=off  set_pwm_outputs_at_switch_out=off  set_pwm_outputs_on_watchdog=off  other_output_channels=[]  initial_other_outputs=[]  final_other_outputs=[]  watchdog_other_outputs=[]  set_other_outputs_at_start=off  set_other_outputs_at_switch_in=off  set_other_outputs_at_terminate=off  set_other_outputs_at_switch_out=off  set_other_outputs_on_watchdog=off
  HIL Read : quarc_library/Data Acquisition/Generic/Immediate I//O/HIL Read  object_name=HIL-1  analog_channels=[0:4]  encoder_channels=[]  digital_channels=[]  other_channels=[1000:1004 3000:3004]  sample_time=qc_get_step_size  active=on  vector_output=off  data_type_mode=Inherit via back propagation  encoder_data_type=double  digital_data_type=boolean
  HIL Set Property : quarc_library/Data Acquisition/Generic/Configuration/HIL Set Property  object_name=HIL-1  property_type=2  property_codes=[128:152]  property_source=2  property_value_num=0  set_at_start=on  sample_time=-1  active=off
      settings: AttributesFormatString=(%<object_name>)  SourceProductName=QUARC Targets
  HIL Write : quarc_library/Data Acquisition/Generic/Immediate I//O/HIL Write  object_name=HIL-1  analog_channels=[]  pwm_channels=[]  digital_channels=[]  other_channels=[1000:1004 11000:11004]  sample_time=-1  active=off  vector_input=off
  Mux : Mux
  Mux1 : Mux
  Mux2 : Mux
  Mux3 : Mux  Inputs=5
  Saturation{,1..4} (5 alike) : Saturate
  Saturation5 : Saturate  UpperLimit=[5*pi/4, pi, 0, 3*pi/4]'  LowerLimit=[-pi/2. 0, -3*pi/4, 0]'
  Saturation6 : Saturate  UpperLimit=[5*pi/4, pi, 0, 3*pi/4]'  LowerLimit=[-pi/2. 0, -3*pi/4, 0]'
  Measured Position (rad) : Outport
  Measured Gripper Position (%) : Outport  Port=2
  Measured Speed (rad/s) : Outport  Port=3
  Measured Gripper Speed(%/s) : Outport  Port=4
  Measured Current (A) : Outport  Port=5
  Measured Gripper Current (A) : Outport  Port=6
  wires:
  Position (rad)/1 -> Saturation5/1
  Demux/2 -> Bias2/1
  Demux/3 -> Bias3/1
  Demux/4 -> Bias4/1
  Bias/1 -> Bias1/1
  Bias1/1 -> HIL Write/1
  Bias2/1 -> Bias6/1
  Bias6/1 -> HIL Write/2
  Bias3/1 -> Bias7/1
  Bias7/1 -> HIL Write/3
  Bias4/1 -> Bias8/1
  Bias8/1 -> HIL Write/4
  Bias5/1 -> Bias9/1
  Bias9/1 -> HIL Write/5
  Gain/1 -> Bias10/1
  PWM (%)/1 -> Demux1/1
  Gripper PWM (%)/1 -> Saturation4/1
  Saturation/1 -> HIL Write/6
  Saturation1/1 -> HIL Write/7
  Saturation2/1 -> HIL Write/8
  Saturation3/1 -> HIL Write/9
  Saturation4/1 -> HIL Write/10
  HIL Read/1 -> Mux/1
  HIL Read/2 -> Mux/2
  HIL Read/3 -> Mux/3
  HIL Read/4 -> Mux/4
  Mux/1 -> Measured Current (A)/1
  HIL Read/5 -> Measured Gripper Current (A)/1
  Bias14/1 -> Bias18/1
  Bias15/1 -> Bias19/1
  Bias17/1 -> Bias21/1
  Bias11/1 -> Bias12/1
  Bias16/1 -> Bias20/1
  HIL Read/6 -> Bias11/1
  HIL Read/7 -> Bias14/1
  HIL Read/8 -> Bias15/1
  HIL Read/9 -> Bias16/1
  HIL Read/10 -> Bias17/1
  Bias21/1 -> Bias13/1
  Bias13/1 -> Gain1/1
  Gain1/1 -> Measured Gripper Position (%)/1
  Mux1/1 -> Saturation6/1
  HIL Read/11 -> Mux2/1
  HIL Read/12 -> Mux2/2
  HIL Read/13 -> Mux2/3
  HIL Read/14 -> Mux2/4
  Mux2/1 -> Measured Speed (rad/s)/1
  HIL Read/15 -> Measured Gripper Speed(%/s)/1
  Constant/1 -> Mux3/1
  Constant1/1 -> Mux3/2
  Constant2/1 -> Mux3/3
  Constant3/1 -> Mux3/4
  Constant4/1 -> Mux3/5
  Mux3/1 -> HIL Set Property/1
  Bias12/1 -> Mux1/1
  Bias18/1 -> Mux1/2
  Bias19/1 -> Mux1/3
  Bias20/1 -> Mux1/4
  Demux1/1 -> Saturation/1
  Demux1/2 -> Saturation1/1
  Demux1/3 -> Saturation2/1
  Demux1/4 -> Saturation3/1
  Demux/1 -> Bias/1
  Saturation5/1 -> Demux/1
  Saturation6/1 -> Measured Position (rad)/1
  Gripper Position (%)/1 -> Gain/1
  Bias10/1 -> Bias5/1

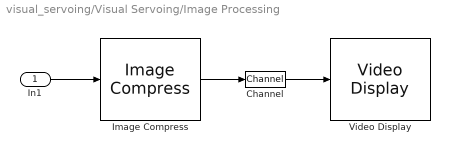
== system visual_servoing/Visual Servoing/Image Processing ==
  In1 : Inport
  Channel : quarc_library/Signal Routing/Channel  channel=0  buffer_size=1
  Image Compress : quarc_library/Image Processing/Generic/Image Compress  algorithm=JPEG  source=Internal dialog parameter  quality=quality  output_dim=-1
  Video Display : quarc_library/Multimedia/Video Display  Tag=visual_servoing_2023a/Visual Servoing/Image Processing/Video Display  sample_time=sample_time  use_hardware=on
  wires:
  Channel/1 -> Video Display/1
  In1/1 -> Image Compress/1
  Image Compress/1 -> Channel/1

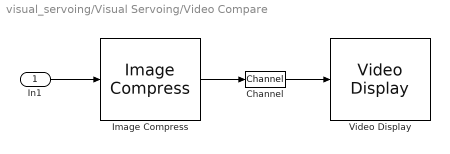
== system visual_servoing/Visual Servoing/Video Compare ==
  In1 : Inport
  Channel : quarc_library/Signal Routing/Channel  channel=1  buffer_size=1
  Image Compress : quarc_library/Image Processing/Generic/Image Compress  algorithm=JPEG  source=Internal dialog parameter  quality=quality  output_dim=-1
  Video Display : quarc_library/Multimedia/Video Display  Tag=visual_servoing_2023a/Visual Servoing/Video Compare/Video Display  sample_time=sample_time  use_hardware=on
  wires:
  Channel/1 -> Video Display/1
  In1/1 -> Image Compress/1
  Image Compress/1 -> Channel/1

== matlab function visual_servoing/QArm Mini/Forward Kinematics ==
  data: theta input; pe output; R0e output; alpha output
function [pe, R0e, alpha] = qArmMiniForwardKinematics(theta)

%% QARM_MINI_FPK
% v 1.0 - 30th March 2025

% REFERENCE: 
% Chapter 3. Forward Kinematics
% Robot Dynamics and Control 
% Spong, Vidyasagar
% 1989

% INPUTS:
% theta   : Alternate joint angles vector 4 x 1

% OUTPUTS:
% pe      : End-effector frame {e} position vector expressed in base frame {0}
% R0e     : rotation matrix from end-effector frame {e} to base frame {0}

%% Manipulator parameters:
L1 = 0.1300;
L2 = 0.1240;
L3 = 0.0230;
L4 = 0.1240;
L5 = 0.1320;

%% Alternate parameters
l1 = L1;
l2 = sqrt(L2^2 + L3^2);
l3 = L4;
l4 = L5;

%% Transformation matrices for all frames:

% T{i-1}{i} = quanser_arm_DH(  a, alpha,  d,     theta );
        T01 = quanser_arm_DH(  0,  pi/2, l1,  theta(1) );
        T12 = quanser_arm_DH( l2,     0,  0,  theta(2) );
        T23 = quanser_arm_DH( l3,     0,  0,  theta(3) );
        T34 = quanser_arm_DH(  0,  pi/2,  0,  theta(4) );
        T4e = quanser_arm_DH(  0,     0, l4,         0 );
        
        T02 = T01*T12;
        T03 = T02*T23;
        T04 = T03*T34;
        T0e = T04*T4e;
        
%% Position of end-effector Transformation

% Extract the Position vector 
p1   = T01(1:3,4);
p2   = T02(1:3,4);
p3   = T03(1:3,4);
p4   = T04(1:3,4);
pe   = T0e(1:3,4);

% Extract the Rotation matrix
R01 = T01(1:3,1:3);
R02 = T02(1:3,1:3);
R03 = T03(1:3,1:3);
R04 = T04(1:3,1:3);
R0e = T0e(1:3,1:3);
alpha = theta(2) + theta(3) + theta(4) - pi/2;
end

function T = quanser_arm_DH(a,alpha,d,theta)

%% QUANSER_ARM_DH
% v 1.0 - 26th March 2019

% REFERENCE: 
% Chapter 3. Forward and Inverse Kinematics
% Robot Modeling and Control 
% Spong, Hutchinson, Vidyasagar
% 2006

% INPUTS:
% a       :   translation  : along : x_{i}   : from : z_{i-1} : to : z_{i}
% alpha   :      rotation  : about : x_{i}   : from : z_{i-1} : to : z_{i}
% d       :   translation  : along : z_{i-1} : from : x_{i-1} : to : x_{i}
% theta   :      rotation  : about : z_{i-1} : from : x_{i-1} : to : x_{i}
% NOTE: Standard DH Parameters

% OUTPUTS:
% T       : transformation                   : from :     {i} : to : {i-1}

%%
% Rotation Transformation about z axis by theta
T_R_z = [cos(theta) -sin(theta) 0 0;
         sin(theta)  cos(theta) 0 0;
                  0           0 1 0;
                  0           0 0 1];
     
% Translation Transformation along z axis by d
T_T_z = [1 0 0 0;
         0 1 0 0;
         0 0 1 d;
         0 0 0 1];

% Translation Transformation along x axis by a
T_T_x = [1 0 0 a;
         0 1 0 0;
         0 0 1 0;
         0 0 0 1];

% Rotation Transformation about x axis by alpha
T_R_x = [1          0           0 0;
         0 cos(alpha) -sin(alpha) 0;
         0 sin(alpha)  cos(alpha) 0;
         0          0           0 1];

% For a transformation FROM frame {i} TO frame {i-1}: A
T = T_R_z*T_T_z*T_T_x*T_R_x;

end

== matlab function visual_servoing/Visual Servoing/MATLAB Function ==
  data: inputImage input; markedImage output; found input; centroid input
function markedImage = fcn(inputImage, found, centroid)
size_im = size(inputImage);
blank_image = uint8(zeros(size_im));
Cross_length = 30; 

if found
    blank_image = inputImage*0.7;
    
    % Horizontal 
    for i = 1:1:Cross_length
    
            blank_image(floor(centroid(1)),floor(centroid(2)-Cross_length/2+i),1:3) = 255;
    end 
    
    % Vertical
    for i = 1:1:Cross_length
            blank_image(centroid(1)-Cross_length/2+i,centroid(2),1:3) = 255;
    end 
    markedImage = blank_image;
else 
    markedImage = inputImage;
end

== matlab function visual_servoing/QArm Mini/MATLAB Function ==
  data: theta input; J output; c output; r output
function [J, c, r] = qarmDifferentialKinematics(theta)

%% QUANSER_ARM_FDK - Returns the Jacobian calculated from analytical eqn.s
% v 1.0 - 9th December 2022

% REFERENCE: 
% Chapter 5. Velocity Kinematics
% Robot Dynamics and Control 
% Spong, Vidyasagar
% 1989

% INPUTS:
% theta   : Alternate joint angles vector 4 x 1

% OUTPUTS:
% J       : Jacobian Matrix

%% Manipulator parameters:
% Link lengths
L1 = 0.1300;
L2 = 0.1240;
L3 = 0.0230;
L4 = 0.1240;
L5 = 0.1320;

% Lambdas
l1 = L1;
l2 = sqrt(L2^2 + L3^2);
l3 = L4;
l4 = L5;

J = eye(4);
J(1,1) = -l2*sin(theta(1))*cos(theta(2)) - l3*sin(theta(1))*cos(theta(2)+theta(3)) - l4*sin(theta(1))*sin(theta(2)+theta(3)+theta(4));
J(1,2) = -l2*cos(theta(1))*sin(theta(2)) - l3*cos(theta(1))*sin(theta(2)+theta(3)) + l4*cos(theta(1))*cos(theta(2)+theta(3)+theta(4));
J(1,3) = -l3*cos(theta(1))*sin(theta(2)+theta(3)) + l4*cos(theta(1))*cos(theta(2)+theta(3)+theta(4));
J(1,4) =  l4*cos(theta(1))*cos(theta(2)+theta(3)+theta(4));
J(2,1) =  l2*cos(theta(1))*cos(theta(2)) + l3*cos(theta(1))*cos(theta(2)+theta(3)) + l4*cos(theta(1))*sin(theta(2)+theta(3)+theta(4));
J(2,2) = -l2*sin(theta(1))*sin(theta(2)) - l3*sin(theta(1))*sin(theta(2)+theta(3)) + l4*sin(theta(1))*sin(theta(2)+theta(3)+theta(4));
J(2,3) = -l3*sin(theta(1))*sin(theta(2)+theta(3)) + l4*sin(theta(1))*sin(theta(2)+theta(3)+theta(4));
J(2,4) =  l4*sin(theta(1))*sin(theta(2)+theta(3)+theta(4));
J(3,1) = 0;
J(3,2) =  l2*cos(theta(2)) + l3*cos(theta(2)+theta(3)) + l4*sin(theta(2)+theta(3)+theta(4));
J(3,3) =  l3*cos(theta(2)+theta(3)) + l4*sin(theta(2)+theta(3)+theta(4));
J(3,4) =  l4*sin(theta(2)+theta(3)+theta(4));
J(4,1) = 0;
J(4,2) = 1;
J(4,3) = 1;
J(4,4) = 1;

% Calculate the condition number and the rank of the Jacobian
c = cond(J);
r = rank(J);
end
